simulink model "systemID"  (R2022a)
settings: Solver=FixedStepAuto  StartTime=0.0  StopTime=60  FixedStep=Ts  RelTol=1e-3
values from neighbouring files (symbols this model uses):
  admittance_ss = c2d(admittance_ss,TsTwin)    [SIDWaveGenerator.m]
  encCountsPerRev = 4096    [initModels_GUI.m]
  encNoisePower = 1e-8    (= 1e-08)    [initModels_GUI.m]
  Kt = 0.943    [initModels_GUI.m]
  N = 3.75    [compareAdmittance.m]    (also in initModels_GUI.m)
  Rpn = 0.5275    [initModels_GUI.m]
  Ts = 1/1000    (= 0.001)    [FOSTWINctrlPost.m]    (also in initModels_GUI.m)
undefined symbols (not defined in the file or in its folder): posFlapAft, posFlapBow, powerI2R, powerMechAft, powerMechBow, powerMechTotal, powerNet, powerStruct, twin2CtrlStruct
libraries: simulink x2
settings Model: Creator=EGI-Z400  LastModifiedBy=jspin
settings SolverCC: ConcurrentTasks=on  PositivePriorityOrder=on
settings DataIOCC: SaveOutput=off  SaveTime=off
settings OptimizationCC: BlockReduction=off  OptimizeBlockIOStorage=off
settings DebuggingCC: TasksWithSamePriorityMsg=none  UnconnectedInputMsg=warning  UnconnectedOutputMsg=warning  UnconnectedLineMsg=warning  ModelReferenceSymbolNameMessage=none
settings HardwareCC: ProdBitPerLong=64  ProdLongLongMode=on  ProdHWDeviceType=Intel->x86-64 (Linux 64)
settings RTWCC: Description=Simulink Real-Time  SystemTargetFile=slrealtime.tlc  TemplateMakefile=slrealtime_default_tmf  RTWVerbose=off  Toolchain=Simulink Real-Time Toolchain  BuildConfiguration=Faster Runs  CodeExecutionProfiling=on  TargetLang=C++  DLArmComputeVersion=19.05

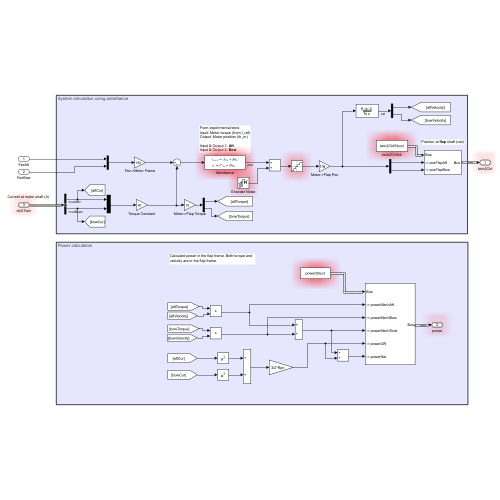
[thumbnail: Simulink's stored preview of the top-level diagram]
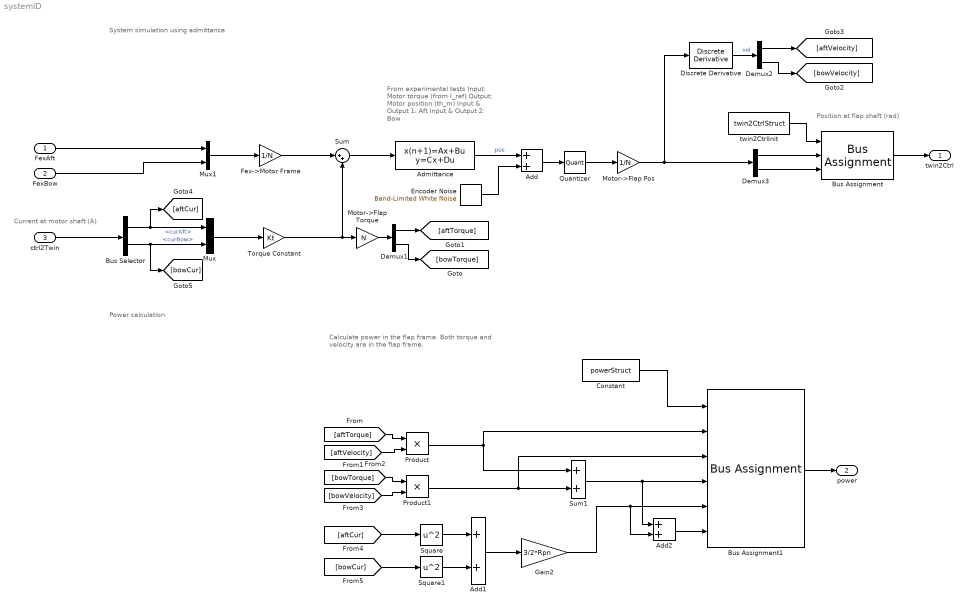
== system systemID ==
  note: Power calculation
  note: System simulation using admittance
  note: Calculate power in the flap frame. Both torque and velocity are in the flap frame.
  note: Current at motor shaft (A)
  note: Position at flap shaft (rad)
  note: From experimental tests
      | Input: Motor torque (from I_ref)
      | Output: Motor position (th_m)
      |
      | Input & Output 1: Aft
      | Input & Output 2: Bow
  FexAft : Inport  Interpolate=off
  FexBow : Inport  Port=2  Interpolate=off
  ctrl2Twin : Inport  Port=3  OutDataTypeStr=Bus: ctrl2TwinBus
  Add : Sum
  Add1 : Sum
  Add2 : Sum
  Admittance : DiscreteStateSpace  A=admittance_ss.A  B=admittance_ss.B  C=admittance_ss.C  D=admittance_ss.D  SampleTime=-1
  Bus Assignment : BusAssignment  AssignedSignals=posFlapAft,posFlapBow
  Bus Assignment1 : BusAssignment  AssignedSignals=powerMechAft,powerMechBow,powerMechTotal,powerI2R,powerNet
  Bus Selector : BusSelector  OutputSignals=curAft,curBow
  Constant : Constant  Value=powerStruct  OutDataTypeStr=Bus: powerBus
  Demux1 : Demux  Outputs=2
  Demux2 : Demux  Outputs=2
  Demux3 : Demux  Outputs=2
  Discrete Derivative : simulink/Discrete/Discrete Derivative  gainval=1.0  ICPrevScaledInput=0.0  OutMin=[]  OutMax=[]  OutDataType=fixdt(1, 16)  OutScaling=2^-10  DoSatur=off
  Encoder Noise : simulink/Sources/Band-Limited White Noise  Cov=[encNoisePower]  Ts=Ts  seed=[23341]
  Fex->Motor Frame : Gain  Gain=1/N
  Gain2 : Gain  Gain=3/2*Rpn
  Motor->Flap Pos : Gain  Gain=1/N
  Motor->Flap Torque : Gain  Gain=N
  Mux : Mux  Inputs=2
  Mux1 : Mux  Inputs=2
  Product : Product
  Product1 : Product
  Quantizer : Quantizer  QuantizationInterval=2*pi/encCountsPerRev
  Square : Math  Operator=square
  Square1 : Math  Operator=square
  Sum : Sum  Inputs=|++  OutDataTypeStr=double
  Sum1 : Sum
  Torque Constant : Gain  Gain=Kt
  twin2CtrlInit : Constant  Value=twin2CtrlStruct  OutDataTypeStr=Bus: twin2CtrlBus
  twin2Ctrl : Outport  OutDataTypeStr=Bus: twin2CtrlBus
  power : Outport  Port=2  OutDataTypeStr=Bus: powerBus
  wires:
  Mux/1 -> Torque Constant/1
  Sum/1 -> Admittance/1
  Mux1/1 -> Fex->Motor Frame/1
  Torque Constant/1 -> Motor->Flap Torque/1, Sum/2
  Discrete Derivative/1 -> Demux2/1  "vel"
  Fex->Motor Frame/1 -> Sum/1
  [aftTorque] -> Product/1
  [aftVelocity] -> Product/2
  [bowTorque] -> Product1/1
  [bowVelocity] -> Product1/2
  Product/1 -> Sum1/1, Bus Assignment1/2
  Product1/1 -> Bus Assignment1/3, Sum1/2
  Demux1/1 -> [aftTorque]
  Demux1/2 -> [bowTorque]
  Demux2/1 -> [aftVelocity]
  Demux2/2 -> [bowVelocity]
  Motor->Flap Torque/1 -> Demux1/1
  Motor->Flap Pos/1 -> Discrete Derivative/1, Demux3/1
  Quantizer/1 -> Motor->Flap Pos/1
  Admittance/1 -> Add/1  "pos"
  Encoder Noise/1 -> Add/2
  Add/1 -> Quantizer/1
  twin2CtrlInit/1 -> Bus Assignment/1
  Demux3/1 -> Bus Assignment/2
  Demux3/2 -> Bus Assignment/3
  Bus Assignment/1 -> twin2Ctrl/1
  FexAft/1 -> Mux1/1
  FexBow/1 -> Mux1/2
  ctrl2Twin/1 -> Bus Selector/1
  Bus Selector/1 -> Mux/1, [aftCur]  "<curAft>"
  Bus Selector/2 -> [bowCur], Mux/2  "<curBow>"
  Constant/1 -> Bus Assignment1/1
  Sum1/1 -> Add2/1, Bus Assignment1/4
  [aftCur] -> Square/1
  [bowCur] -> Square1/1
  Square/1 -> Add1/1
  Square1/1 -> Add1/2
  Add1/1 -> Gain2/1
  Gain2/1 -> Add2/2, Bus Assignment1/5
  Add2/1 -> Bus Assignment1/6
  Bus Assignment1/1 -> power/1
